simulink model "timedelay"  (R2014a)
settings: Solver=ode45  StartTime=0.0  StopTime=10.0  RelTol=1e-3
values from neighbouring files (symbols this model uses):
  a = 21    [blackbox_step_graph.m]    (also in working.mat)
  tau = 0.0033    [working.mat]
settings Model: Creator=gabriellemerritt  LastModifiedBy=gabriellemerritt

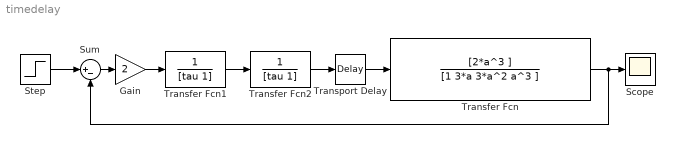
== system timedelay ==
  Gain : Gain  Gain=2
  Scope : Scope
      settings: TimeRange=3  YMin=0  YMax=1.8  SaveName=ScopeData2
  Step : Step  SampleTime=0
  Sum : Sum  Inputs=|+-
  Transfer Fcn : TransferFcn  Numerator=[2*a^3 ]  Denominator=[1 3*a 3*a^2 a^3 ]
  Transfer Fcn1 : TransferFcn  Denominator=[tau 1]
  Transfer Fcn2 : TransferFcn  Denominator=[tau 1]
  Transport Delay : TransportDelay  DelayTime=.01
  wires:
  Transfer Fcn/1 -> Scope/1, Sum/2
  Sum/1 -> Gain/1
  Step/1 -> Sum/1
  Gain/1 -> Transfer Fcn1/1
  Transfer Fcn1/1 -> Transfer Fcn2/1
  Transfer Fcn2/1 -> Transport Delay/1
  Transport Delay/1 -> Transfer Fcn/1
